simulink model "train"  (R2022a)
settings: Solver=ode4  StartTime=0.0  StopTime=30  FixedStep=0.001  RelTol=1e-3
values from neighbouring files (symbols this model uses):
  F = 1    [setup.m]
  g = 9.8    [setup.m]
  k = 1    [setup.m]
  M1 = 0.5    [setup.m]
  M2 = 1    [setup.m]
  mu = 0.02    [setup.m]
settings Model: Creator=stakk  LastModifiedBy=stakk

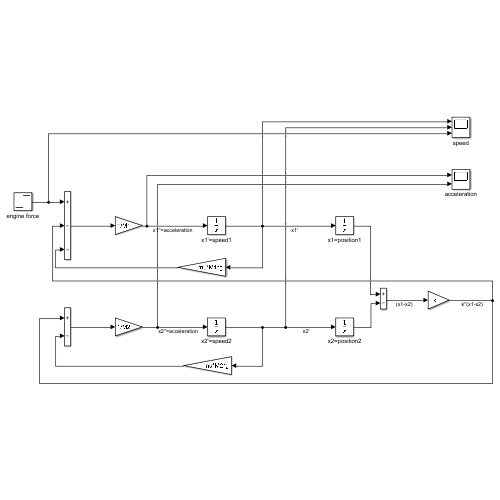
[thumbnail: Simulink's stored preview of the top-level diagram]
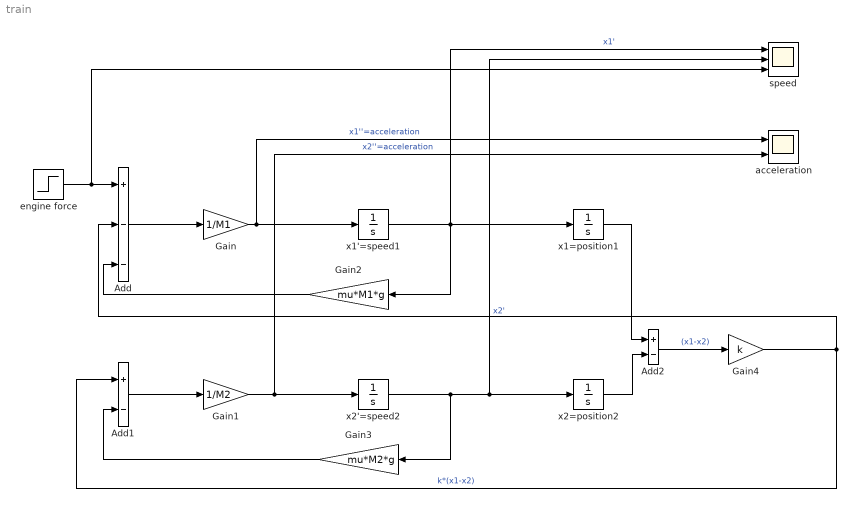
== system train ==
  Add : Sum  Inputs=+--
  Add1 : Sum  Inputs=+-
  Add2 : Sum  Inputs=+-
  Gain : Gain  Gain=1/M1
  Gain1 : Gain  Gain=1/M2
  Gain2 : Gain  Gain=mu*M1*g
  Gain3 : Gain  Gain=mu*M2*g
  Gain4 : Gain  Gain=k
  acceleration : Scope  NumInputPorts=2
  engine force : Step  After=F  SampleTime=0
  speed : Scope  NumInputPorts=3
  x1'=speed1 : Integrator
  x1=position1 : Integrator
  x2'=speed2 : Integrator
  x2=position2 : Integrator
  wires:
  x1'=speed1/1 -> speed/1, Gain2/1, x1=position1/1  "x1'"
  Add/1 -> Gain/1
  Gain/1 -> acceleration/1, x1'=speed1/1  "x1''=acceleration"
  engine force/1 -> speed/3, Add/1
  Gain2/1 -> Add/3
  Gain3/1 -> Add1/2
  x2'=speed2/1 -> Gain3/1, speed/2, x2=position2/1  "x2'"
  Gain1/1 -> acceleration/2, x2'=speed2/1  "x2''=acceleration"
  Add1/1 -> Gain1/1
  x1=position1/1 -> Add2/1
  x2=position2/1 -> Add2/2
  Add2/1 -> Gain4/1  "(x1-x2)"
  Gain4/1 -> Add1/1, Add/2  "k*(x1-x2)"
